simulink model "generic_truck"  (R2025a)
settings: Solver=VariableStepAuto  StartTime=0.0  StopTime=600  FixedStep=0.01  MaxStep=0.001  RelTol=1e-3  EnableMultiTasking=on
libraries: TruckMaker4SL x205, simulink x1
(part 2 of 9)

== system generic_truck/TruckMaker/IPG Vehicle/PowerTrain ==
  note: When replacing the entire powertrain,
      | be sure to disable the IPG powertrain model by using the powertrain
      | model 'Model Manager off' in the vehicle GUI.
  note: <Your model here>
  Sync_In : Inport
  Vhcl.Wheel.PT : Inport  Port=2
  VhclCtrl.PT : Inport  Port=3
  BusCreator : BusCreator  Inputs=99
  Demux : Demux  Outputs=99
      settings: DisplayOption=none
  Gain : Gain
  PowerTrain : S-Function  FunctionName=TM_Sfun  Parameters='PowerTrain'  SFunctionDeploymentMode=off  EnableBusSupport=off
  PowerTrainUpd : S-Function  FunctionName=TM_Sfun  Parameters='PowerTrainUpd'  SFunctionDeploymentMode=off  EnableBusSupport=off
  Sum : Sum  Inputs=|++
  Sync_Out : Outport  VectorParamsAs1DForOutWhenUnconnected=off
  WRR_Trq-drive : Outport  Port=2
  wires:
  Demux/97 -> BusCreator/97  "PT IF WRR4 Trq_Supp2WC"
  Demux/95 -> BusCreator/95  "PT IF WRR4 Trq_B2W"
  Demux/92 -> BusCreator/92  "PT IF WRL4 Trq_BrakeReg_max"
  Demux/88 -> BusCreator/88  "PT IF WRL4 Trq_B2W"
  Demux/89 -> BusCreator/89  "PT IF WRL4 Trq_Drive"
  Demux/86 -> BusCreator/86  "PT IF WRL4 rot"
  Demux/91 -> BusCreator/91  "PT IF WRL4 Trq_BrakeReg"
  Demux/84 -> BusCreator/84  "PT IF WRR3 Trq_BrakeReg"
  Demux/83 -> BusCreator/83  "PT IF WRR3 Trq_Supp2WC"
  Demux/82 -> BusCreator/82  "PT IF WRR3 Trq_Drive"
  Demux/78 -> BusCreator/78  "PT IF WRL3 Trq_BrakeReg_max"
  Demux/87 -> BusCreator/87  "PT IF WRL4 rotv"
  Demux/77 -> BusCreator/77  "PT IF WRL3 Trq_BrakeReg"
  Demux/75 -> BusCreator/75  "PT IF WRL3 Trq_Drive"
  Demux/73 -> BusCreator/73  "PT IF WRL3 rotv"
  Demux/72 -> BusCreator/72  "PT IF WRL3 rot"
  Demux/71 -> BusCreator/71  "PT IF WFR2 Trq_BrakeReg_max"
  Demux/70 -> BusCreator/70  "PT IF WFR2 Trq_BrakeReg"
  Demux/67 -> BusCreator/67  "PT IF WFR2 Trq_B2W"
  Demux/66 -> BusCreator/66  "PT IF WFR2 rotv"
  Demux/80 -> BusCreator/80  "PT IF WRR3 rotv"
  Demux/65 -> BusCreator/65  "PT IF WFR2 rot"
  Demux/76 -> BusCreator/76  "PT IF WRL3 Trq_Supp2WC"
  Demux/63 -> BusCreator/63  "PT IF WFL2 Trq_BrakeReg"
  Demux/74 -> BusCreator/74  "PT IF WRL3 Trq_B2W"
  Demux/69 -> BusCreator/69  "PT IF WFR2 Trq_Supp2WC"
  Demux/58 -> BusCreator/58  "PT IF WFL2 rot"
  Demux/68 -> BusCreator/68  "PT IF WFR2 Trq_Drive"
  Demux/56 -> BusCreator/56  "PT IF WRR2 Trq_BrakeReg"
  Demux/61 -> BusCreator/61  "PT IF WFL2 Trq_Drive"
  Demux/24 -> BusCreator/24  "PT IF WFR rotv"
  BusCreator/1 -> PowerTrainUpd/2
  Demux/20 -> BusCreator/20  "PT IF WFL Trq_Supp2WC"
  Demux/13 -> BusCreator/13  "PT IF Trq_Supp2BdyEng x"
  Demux/99 -> BusCreator/99  "PT IF WRR4 Trq_BrakeReg_max"
  Demux/19 -> BusCreator/19  "PT IF WFL Trq_Drive"
  Demux/33 -> Sum/1, BusCreator/33  "PT IF WRL Trq_Drive"
  Demux/29 -> BusCreator/29  "PT IF WFR Trq_BrakeReg_max"
  Demux/64 -> BusCreator/64  "PT IF WFL2 Trq_BrakeReg_max"
  Demux/57 -> BusCreator/57  "PT IF WRR2 Trq_BrakeReg_max"
  Demux/42 -> BusCreator/42  "PT IF WRR Trq_BrakeReg"
  Demux/16 -> BusCreator/16  "PT IF WFL rot"
  Demux/26 -> BusCreator/26  "PT IF WFR Trq_Drive"
  PowerTrainUpd/1 -> Sync_Out/1
  Demux/93 -> BusCreator/93  "PT IF WRR4 rot"
  Demux/79 -> BusCreator/79  "PT IF WRR3 rot"
  Demux/37 -> BusCreator/37  "PT IF WRR rot"
  Demux/15 -> BusCreator/15  "PT IF DL_iDiff_mean"
  Demux/4 -> BusCreator/4  "PT IF OperationError"
  Demux/59 -> BusCreator/59  "PT IF WFL2 rotv"
  Demux/11 -> BusCreator/11  "PT IF Trq_Supp2Bdy1B y"
  Demux/90 -> BusCreator/90  "PT IF WRL4 Trq_Supp2WC"
  Demux/9 -> BusCreator/9  "PT IF Trq_Supp2Bdy1 z"
  Demux/1 -> BusCreator/1  "PT IF Ignition"
  Demux/98 -> BusCreator/98  "PT IF WRR4 Trq_BrakeReg"
  Demux/17 -> BusCreator/17  "PT IF WFL rotv"
  Sync_In/1 -> PowerTrain/1
  PowerTrain/2 -> Demux/1
  Vhcl.Wheel.PT/1 -> PowerTrain/2
  Demux/14 -> BusCreator/14  "PT IF Trq_Supp2BdyEng y"
  Demux/8 -> BusCreator/8  "PT IF Trq_Supp2Bdy1 y"
  PowerTrain/1 -> PowerTrainUpd/1  "Sync"
  Demux/40 -> Sum/2, BusCreator/40  "PT IF WRR Trq_Drive"
  Demux/12 -> BusCreator/12  "PT IF Trq_Supp2Bdy1B z"
  Demux/2 -> BusCreator/2  "PT IF SelectorCtrl"
  Demux/22 -> BusCreator/22  "PT IF WFL Trq_BrakeReg_max"
  Demux/3 -> BusCreator/3  "PT IF OperationState"
  Demux/10 -> BusCreator/10  "PT IF Trq_Supp2Bdy1B x"
  Demux/18 -> BusCreator/18  "PT IF WFL Trq_B2W"
  Demux/6 -> BusCreator/6  "PT IF Engine_rotv"
  Demux/5 -> BusCreator/5  "PT IF GearNo"
  Demux/27 -> BusCreator/27  "PT IF WFR Trq_Supp2WC"
  Demux/52 -> BusCreator/52  "PT IF WRR2 rotv"
  Demux/28 -> BusCreator/28  "PT IF WFR Trq_BrakeReg"
  Demux/41 -> BusCreator/41  "PT IF WRR Trq_Supp2WC"
  Demux/31 -> BusCreator/31  "PT IF WRL rotv"
  Demux/94 -> BusCreator/94  "PT IF WRR4 rotv"
  Demux/55 -> BusCreator/55  "PT IF WRR2 Trq_Supp2WC"
  Demux/32 -> BusCreator/32  "PT IF WRL Trq_B2W"
  Demux/35 -> BusCreator/35  "PT IF WRL Trq_BrakeReg"
  Demux/25 -> BusCreator/25  "PT IF WFR Trq_B2W"
  Demux/39 -> BusCreator/39  "PT IF WRR Trq_B2W"
  Demux/38 -> BusCreator/38  "PT IF WRR rotv"
  Demux/21 -> BusCreator/21  "PT IF WFL Trq_BrakeReg"
  VhclCtrl.PT/1 -> PowerTrain/3
  Demux/36 -> BusCreator/36  "PT IF WRL Trq_BrakeReg_max"
  Demux/60 -> BusCreator/60  "PT IF WFL2 Trq_B2W"
  Demux/43 -> BusCreator/43  "PT IF WRR Trq_BrakeReg_max"
  Demux/44 -> BusCreator/44  "PT IF WRL2 rot"
  Demux/81 -> BusCreator/81  "PT IF WRR3 Trq_B2W"
  Demux/30 -> BusCreator/30  "PT IF WRL rot"
  Demux/45 -> BusCreator/45  "PT IF WRL2 rotv"
  Demux/23 -> BusCreator/23  "PT IF WFR rot"
  Demux/46 -> BusCreator/46  "PT IF WRL2 Trq_B2W"
  Demux/96 -> BusCreator/96  "PT IF WRR4 Trq_Drive"
  Demux/54 -> BusCreator/54  "PT IF WRR2 Trq_Drive"
  Demux/85 -> BusCreator/85  "PT IF WRR3 Trq_BrakeReg_max"
  Demux/47 -> BusCreator/47  "PT IF WRL2 Trq_Drive"
  Demux/62 -> BusCreator/62  "PT IF WFL2 Trq_Supp2WC"
  Demux/7 -> BusCreator/7  "PT IF Trq_Supp2Bdy1 x"
  Demux/48 -> BusCreator/48  "PT IF WRL2 Trq_Supp2WC"
  Demux/34 -> BusCreator/34  "PT IF WRL Trq_Supp2WC"
  Demux/49 -> BusCreator/49  "PT IF WRL2 Trq_BrakeReg"
  Demux/50 -> BusCreator/50  "PT IF WRL2 Trq_BrakeReg_max"
  Demux/51 -> BusCreator/51  "PT IF WRR2 rot"
  Demux/53 -> BusCreator/53  "PT IF WRR2 Trq_B2W"
  Sum/1 -> Gain/1
  Gain/1 -> WRR_Trq-drive/1

== system generic_truck/TruckMaker/Subsystem1/Measurements from IMU ==
  Acc_x : TruckMaker4SL/Read CM Dict  xname=Sensor.Inertial.Vhcl.VchBdy.Acc_B.x  xsync=off  xstime=Continuous
      settings: SourceProductName=TruckMaker4SL
  Acc_x1 : TruckMaker4SL/Read CM Dict  xname=Vhcl.RL.rotv  xsync=off  xstime=Continuous
      settings: SourceProductName=TruckMaker4SL
  Acc_x2 : TruckMaker4SL/Read CM Dict  xname=Vhcl.RR.rotv  xsync=off  xstime=Continuous
      settings: SourceProductName=TruckMaker4SL
  Acc_x3 : TruckMaker4SL/Read CM Dict  xname=Tr.WheelSpd_ML  xsync=off  xstime=Continuous
      settings: SourceProductName=TruckMaker4SL
  Acc_x4 : TruckMaker4SL/Read CM Dict  xname=Tr.WheelSpd_MR  xsync=off  xstime=Continuous
      settings: SourceProductName=TruckMaker4SL
  Acc_y : TruckMaker4SL/Read CM Dict  xname=Sensor.Inertial.Vhcl.VchBdy.Acc_B.y  xsync=off  xstime=Continuous
      settings: SourceProductName=TruckMaker4SL
  Omega_z : TruckMaker4SL/Read CM Dict  xname=Sensor.Inertial.Vhcl.VchBdy.Omega_B.z  xsync=off  xstime=Continuous
      settings: SourceProductName=TruckMaker4SL
  Vel_x : TruckMaker4SL/Read CM Dict  xname=Sensor.Inertial.Vhcl.VchBdy.Vel_B.x  xsync=off  xstime=Continuous
      settings: SourceProductName=TruckMaker4SL
  Vel_y : TruckMaker4SL/Read CM Dict  xname=Sensor.Inertial.Vhcl.VchBdy.Vel_B.y  xsync=off  xstime=Continuous
      settings: SourceProductName=TruckMaker4SL
  acc_x : Outport
  acc_y : Outport  Port=2
  vel_x : Outport  Port=3
  vel_y : Outport  Port=4
  wz : Outport  Port=5
  omega_rl : Outport  Port=6
  omega_rr : Outport  Port=7
  omega_tr_ML : Outport  Port=8
  omega_tr_MR : Outport  Port=9
  wires:
  Omega_z/1 -> wz/1
  Vel_x/1 -> vel_x/1
  Vel_y/1 -> vel_y/1
  Acc_x/1 -> acc_x/1
  Acc_y/1 -> acc_y/1
  Acc_x2/1 -> omega_rr/1
  Acc_x1/1 -> omega_rl/1
  Acc_x3/1 -> omega_tr_ML/1
  Acc_x4/1 -> omega_tr_MR/1

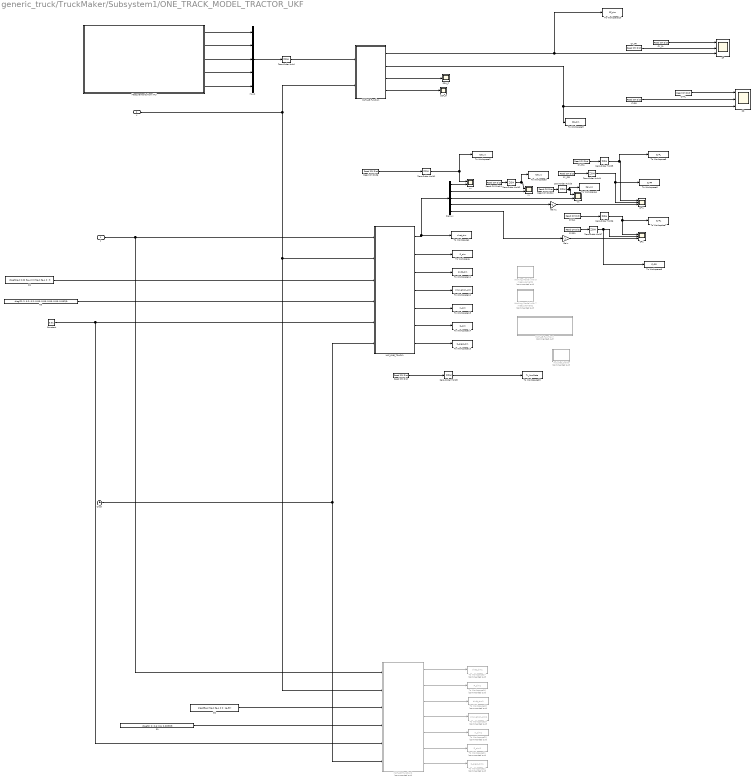
== system generic_truck/TruckMaker/Subsystem1/ONE_TRACK_MODEL_TRACTOR_UKF ==
  z : Inport
  u : Inport  Port=2
  "CF " : Scope  NumInputPorts=3
      settings: ActiveDisplayYMinimum=-12.263034323337607  ActiveDisplayYMaximum=-4.9489164501428942  DataLoggingVariableName=ScopeData23
  CF 1 : Scope  NumInputPorts=3
      settings: ActiveDisplayYMinimum=-10.797860186662938  ActiveDisplayYMaximum=-3.0037046797887497  DataLoggingVariableName=ScopeData30
  CR : Scope  NumInputPorts=3
      settings: ActiveDisplayYMinimum=-11.701585356235972  ActiveDisplayYMaximum=4.5045535239425494  DataLoggingVariableName=ScopeData24
  CR1 : Scope  NumInputPorts=3
      settings: ActiveDisplayYMinimum=-13.474282112558932  ActiveDisplayYMaximum=-8.0648262356989679  DataLoggingVariableName=ScopeData31
  CYRL : TruckMaker4SL/Read CM Dict  xname=CyRL  xsync=off  xstime=Continuous
      settings: SourceProductName=TruckMaker4SL
  CYRL1 : TruckMaker4SL/Read CM Dict  xname=CyRL  xsync=off  xstime=Continuous
      settings: SourceProductName=TruckMaker4SL
  CYRR : TruckMaker4SL/Read CM Dict  xname=CyRR  xsync=off  xstime=Continuous
      settings: SourceProductName=TruckMaker4SL
  CYRR1 : TruckMaker4SL/Read CM Dict  xname=CyRR  xsync=off  xstime=Continuous
      settings: SourceProductName=TruckMaker4SL
  CY_FL : TruckMaker4SL/Read CM Dict  xname=CyFL  xsync=off  xstime=Continuous
      settings: SourceProductName=TruckMaker4SL
  CY_FL1 : TruckMaker4SL/Read CM Dict  xname=CyFL  xsync=off  xstime=Continuous
      settings: SourceProductName=TruckMaker4SL
  CY_FR : TruckMaker4SL/Read CM Dict  xname=CyFR  xsync=off  xstime=Continuous
      settings: SourceProductName=TruckMaker4SL
  CY_FR1 : TruckMaker4SL/Read CM Dict  xname=CyFR  xsync=off  xstime=Continuous
      settings: SourceProductName=TruckMaker4SL
  Clock : Clock
  Constant : Constant  Value=0.01
  Demux : Demux  Outputs=5
  Gain : Gain  Gain=-1
  Gain1 : Gain  Gain=-1
  "Included_trailer " : MATLAB Function  Commented=on  TreatAsAtomicUnit=on
  MATLAB Function : MATLAB Function  TreatAsAtomicUnit=on
  MATLAB Function1 : MATLAB Function  Commented=on  TreatAsAtomicUnit=on
  MATLAB Function2 : MATLAB Function  Commented=on  TreatAsAtomicUnit=on  SystemSampleTime=0.01
  Measurements from IMU : Subsystem  Description=Measurements from IMU Mounted in Vhcl position (3.6; 0.0;1.0)
  Mux2 : Mux  Inputs=5
  Q1 : Constant  Value="diag([2e-2 0.02 3e-4 0 0 5e-2 3e-4 0  ]);"
  Q2 : Constant  Value="diag([5e-2 5e-2 3e-4 0 0  1e-3]);"
  R1 : Constant  Value=diag([2; 2; 0.6; 0.6; 0.005])/3;
  R3 : Constant  Value=diag([2; 2; 0.2; 0.2; 0.05; 0.05; 0.05; 0.05; 0.05])/3;
  Read CM Dict : TruckMaker4SL/Read CM Dict  xname=Tr.YawVel  xsync=off  xstime=Continuous
      settings: SourceProductName=TruckMaker4SL
  Read CM Dict11 : TruckMaker4SL/Read CM Dict  xname=Car.vy  xsync=off  xstime=Continuous
      settings: SourceProductName=TruckMaker4SL
  Read CM Dict12 : TruckMaker4SL/Read CM Dict  xname=Car.YawRate  xsync=off  xstime=Continuous
      settings: SourceProductName=TruckMaker4SL
  Read CM Dict6 : TruckMaker4SL/Read CM Dict  xname=Car.vx  xsync=off  xstime=Continuous
      settings: SourceProductName=TruckMaker4SL
  SSA_F : Scope
      settings: ActiveDisplayYMinimum=-0.046315426334515186  ActiveDisplayYMaximum=0.00321973029301955  DataLoggingVariableName=ScopeData25
  SSA_R : Scope
      settings: ActiveDisplayYMinimum=19.809904868748255  ActiveDisplayYMaximum=19.861105266179973  DataLoggingVariableName=ScopeData26
  To Workspace : ToWorkspace  VariableName=P_sim  SaveFormat=Timeseries  SampleTime=-1
  To Workspace1 : ToWorkspace  VariableName=xhat_sim  SaveFormat=Timeseries  SampleTime=-1
  To Workspace10 : ToWorkspace  VariableName=CF_sim  SaveFormat=Timeseries  SampleTime=-1
  To Workspace11 : ToWorkspace  VariableName=dxdt_sim  SaveFormat=Timeseries  SampleTime=-1
  To Workspace12 : ToWorkspace  VariableName=innovation_sim  SaveFormat=Timeseries  SampleTime=-1
  To Workspace13 : ToWorkspace  VariableName=K_sim  SaveFormat=Timeseries  SampleTime=-1
  To Workspace14 : ToWorkspace  VariableName=S_sim  SaveFormat=Timeseries  SampleTime=-1
  To Workspace15 : ToWorkspace  VariableName=Z_pred_sim  SaveFormat=Timeseries  SampleTime=-1
  To Workspace16 : ToWorkspace  Commented=on  VariableName=P_sim1  SaveFormat=Timeseries  SampleTime=-1
  To Workspace17 : ToWorkspace  Commented=on  VariableName=xhat_sim1  SaveFormat=Timeseries  SampleTime=-1
  To Workspace18 : ToWorkspace  Commented=on  VariableName=dxdt_sim1  SaveFormat=Timeseries  SampleTime=-1
  To Workspace19 : ToWorkspace  Commented=on  VariableName=innovation_sim1  SaveFormat=Timeseries  SampleTime=-1
  To Workspace2 : ToWorkspace  VariableName=Car_vx  SaveFormat=Timeseries  SampleTime=-1
  To Workspace20 : ToWorkspace  Commented=on  VariableName=K_sim1  SaveFormat=Timeseries  SampleTime=-1
  To Workspace21 : ToWorkspace  Commented=on  VariableName=S_sim1  SaveFormat=Timeseries  SampleTime=-1
  To Workspace22 : ToWorkspace  Commented=on  VariableName=Z_pred_sim1  SaveFormat=Timeseries  SampleTime=-1
  To Workspace23 : ToWorkspace  VariableName=Tr_YawRate  SaveFormat=Timeseries  SampleTime=-1
  To Workspace3 : ToWorkspace  VariableName=Car_vy  SaveFormat=Timeseries  SampleTime=-1
  To Workspace4 : ToWorkspace  VariableName=Car_wz  SaveFormat=Timeseries  SampleTime=-1
  To Workspace5 : ToWorkspace  VariableName=CyFL  SaveFormat=Timeseries  SampleTime=-1
  To Workspace6 : ToWorkspace  VariableName=CyFR  SaveFormat=Timeseries  SampleTime=-1
  To Workspace7 : ToWorkspace  VariableName=CyRL  SaveFormat=Timeseries  SampleTime=-1
  To Workspace8 : ToWorkspace  VariableName=CyRR  SaveFormat=Timeseries  SampleTime=-1
  To Workspace9 : ToWorkspace  VariableName=CR_sim  SaveFormat=Timeseries  SampleTime=-1
  UKF_ONE_TRACK1 : MATLAB Function  TreatAsAtomicUnit=on  SystemSampleTime=0.01
  "Working Model with 5 measurements " : MATLAB Function  Commented=on  TreatAsAtomicUnit=on
  Working Model with 7 measurements : MATLAB Function  Commented=on  TreatAsAtomicUnit=on
  Zero-Order Hold{,1..8} (9 alike) : ZeroOrderHold  SampleTime=0.01
  vx : Scope  NumInputPorts=2
      settings: ActiveDisplayYMinimum=15.532965030483135  ActiveDisplayYMaximum=19.510688761225374  DataLoggingVariableName=ScopeData34
  vy : Scope  NumInputPorts=2
      settings: ActiveDisplayYMinimum=-0.016234882238860611  ActiveDisplayYMaximum=0.084455127817541567  DataLoggingVariableName=ScopeData35
  wz : Scope  NumInputPorts=2
      settings: ActiveDisplayYMinimum=-0.21237399330212148  ActiveDisplayYMaximum=0.50990512712526215  DataLoggingVariableName=ScopeData36
  wires:
  MATLAB Function/1(Cf) -> To Workspace10/1, "CF "/3  "Cmptd_Cf"
  Read CM Dict6/1 -> Zero-Order Hold1/1
  CY_FR1/1 -> Zero-Order Hold4/1  "CyFR"
  Demux/1 -> vx/2  "est_vx"
  UKF_ONE_TRACK1/2(P) -> To Workspace/1
  UKF_ONE_TRACK1/1(xhat) -> Demux/1, To Workspace1/1  "State_estimates"
  R3/1 -> UKF_ONE_TRACK1/4(R)
  CYRL1/1 -> Zero-Order Hold6/1  "CyRL"
  Gain/1 -> CR1/3  "est_CR"
  CYRL/1 -> CR/1  "CyRL"
  Constant/1 -> MATLAB Function2/5(Ts), UKF_ONE_TRACK1/5(Ts)
  Read CM Dict12/1 -> Zero-Order Hold3/1
  MATLAB Function/4(alpha_r) -> SSA_R/1
  CYRR1/1 -> Zero-Order Hold7/1  "CyRR"
  CYRR/1 -> CR/2  "CyRR"
  Demux/2 -> vy/2  "est_vy"
  MATLAB Function/2(Cr) -> To Workspace9/1, CR/3  "cmptd_R"
  CY_FL1/1 -> Zero-Order Hold5/1  "CyFL"
  Read CM Dict11/1 -> Zero-Order Hold2/1
  Demux/5 -> Gain/1  "cmptd_R"
  CY_FL/1 -> "CF "/1  "CyFL"
  Demux/3 -> wz/2  "est_wz"
  CY_FR/1 -> "CF "/2  "CyFR"
  MATLAB Function/3(alpha_f) -> SSA_F/1
  Demux/4 -> Gain1/1  "Cmptd_Cf"
  Gain1/1 -> CF 1/3  "Est_CF"
  UKF_ONE_TRACK1/3(dxdt) -> To Workspace11/1
  Q1/1 -> UKF_ONE_TRACK1/3(Q)
  u/1 -> MATLAB Function/2(u), MATLAB Function2/2(u), UKF_ONE_TRACK1/2(u)
  UKF_ONE_TRACK1/4(innovation) -> To Workspace12/1
  UKF_ONE_TRACK1/5(K_out) -> To Workspace13/1
  UKF_ONE_TRACK1/6(S_out) -> To Workspace14/1
  UKF_ONE_TRACK1/7(z_pred_out) -> To Workspace15/1
  z/1 -> MATLAB Function2/1(z), UKF_ONE_TRACK1/1(z)
  Measurements from IMU/1(acc_x) -> Mux2/1
  Measurements from IMU/4(vel_y) -> Mux2/4
  Measurements from IMU/3(vel_x) -> Mux2/3
  Mux2/1 -> Zero-Order Hold/1
  Measurements from IMU/2(acc_y) -> Mux2/2
  Measurements from IMU/5(wz) -> Mux2/5
  Clock/1 -> UKF_ONE_TRACK1/6(data), MATLAB Function2/6(data)
  MATLAB Function2/7(z_pred_out) -> To Workspace22/1
  MATLAB Function2/6(S_out) -> To Workspace21/1
  MATLAB Function2/5(K_out) -> To Workspace20/1
  MATLAB Function2/4(innovation) -> To Workspace19/1
  MATLAB Function2/3(dxdt) -> To Workspace18/1
  MATLAB Function2/1(xhat) -> To Workspace17/1  "State_estimates"
  MATLAB Function2/2(P) -> To Workspace16/1
  R1/1 -> MATLAB Function2/4(R)
  Q2/1 -> MATLAB Function2/3(Q)
  Zero-Order Hold/1 -> MATLAB Function/1(z)
  Zero-Order Hold1/1 -> To Workspace2/1, vx/1
  Zero-Order Hold2/1 -> To Workspace3/1, vy/1
  Zero-Order Hold3/1 -> To Workspace4/1, wz/1
  Zero-Order Hold4/1 -> To Workspace6/1, CF 1/2
  Zero-Order Hold5/1 -> To Workspace5/1, CF 1/1
  Zero-Order Hold6/1 -> To Workspace7/1, CR1/1
  Zero-Order Hold7/1 -> To Workspace8/1, CR1/2
  Read CM Dict/1 -> Zero-Order Hold8/1
  Zero-Order Hold8/1 -> To Workspace23/1

== system generic_truck/TruckMaker/Subsystem1/Subsystem ==
  Ackerman Angle : Subsystem  Commented=on
  Average Steering Angle : Subsystem
  FXh : TruckMaker4SL/Read CM Dict  xname=Tr.Hitch.Frc2Tr.x_1  xsync=off  xstime=Continuous
      settings: SourceProductName=TruckMaker4SL
  FYh : TruckMaker4SL/Read CM Dict  xname=Tr.Hitch.Frc2Tr.y_1  xsync=off  xstime=Continuous
      settings: SourceProductName=TruckMaker4SL
  Trq_RL : TruckMaker4SL/Read CM Dict  xname=Vhcl.RL.Trq_Drive  xsync=off  xstime=Continuous
      settings: SourceProductName=TruckMaker4SL
  Trq_RR : TruckMaker4SL/Read CM Dict  xname=Vhcl.RR.Trq_Drive  xsync=off  xstime=Continuous
      settings: SourceProductName=TruckMaker4SL
  "Average_steering " : Outport
  Trq_T2W_RL : Outport  Port=2
  Trq_T2W_RR : Outport  Port=3
  FXH : Outport  Port=4
  FYH : Outport  Port=5
  wires:
  Trq_RL/1 -> Trq_T2W_RL/1
  Trq_RR/1 -> Trq_T2W_RR/1
  Average Steering Angle/1("Average_steering ") -> "Average_steering "/1
  FXh/1 -> FXH/1
  FYh/1 -> FYH/1

== system generic_truck/TruckMaker/Subsystem1/Subsystem_Noisey Measurements ==
  Acc_x : TruckMaker4SL/Read CM Dict  xname=Vhcl.RL.rotv  xsync=off  xstime=Continuous
      settings: SourceProductName=TruckMaker4SL
  Acc_x1 : TruckMaker4SL/Read CM Dict  xname=Vhcl.RR.rotv  xsync=off  xstime=Continuous
      settings: SourceProductName=TruckMaker4SL
  Acc_x3 : TruckMaker4SL/Read CM Dict  xname=Tr.WheelSpd_ML  xsync=off  xstime=Continuous
      settings: SourceProductName=TruckMaker4SL
  Acc_x4 : TruckMaker4SL/Read CM Dict  xname=Tr.WheelSpd_MR  xsync=off  xstime=Continuous
      settings: SourceProductName=TruckMaker4SL
  Demux : Demux  Outputs=2
  Demux1 : Demux  Outputs=2
  Demux2 : Demux  Outputs=2
  Demux3 : Demux  Outputs=1
  MATLAB Function : MATLAB Function  TreatAsAtomicUnit=on
  MATLAB Function1 : MATLAB Function  TreatAsAtomicUnit=on
  MATLAB Function2 : MATLAB Function  TreatAsAtomicUnit=on
  MATLAB Function3 : MATLAB Function  TreatAsAtomicUnit=on
  Measurements from IMU : Subsystem  Description=Measurements from IMU Mounted in Vhcl position (3.6; 0.0;1.0)
  Mux : Mux  Inputs=3
  Mux1 : Mux  Inputs=3
  Mux2 : Mux  Inputs=5
  Mux3 : Mux  Inputs=3
  Mux5 : Mux  Inputs=2
  Mux6 : Mux  Inputs=2
  Scope : Scope
      settings: ActiveDisplayYMinimum=-5.6580655588196418  ActiveDisplayYMaximum=20.488387754127984  DataLoggingVariableName=ScopeData37
  Out1 : Outport
  wires:
  Mux1/1 -> MATLAB Function2/1(truth)
  Mux2/1 -> Scope/1, Out1/1
  Measurements from IMU/3(acc_z) -> Mux3/3
  Measurements from IMU/2(acc_y) -> Mux3/2
  Measurements from IMU/1(acc_x) -> Mux3/1
  Mux3/1 -> MATLAB Function1/1(acc_true)
  Measurements from IMU/4(vel_x) -> Mux1/1
  Measurements from IMU/5(vel_y) -> Mux1/2
  Measurements from IMU/6(vel_z) -> Mux1/3
  Mux/1 -> MATLAB Function/1(gyro_true)
  Measurements from IMU/7(wx) -> Mux/1
  Measurements from IMU/8(wy) -> Mux/2
  Measurements from IMU/9(wz) -> Mux/3
  Demux/1 -> Mux2/1
  Demux1/1 -> Mux2/2
  Demux2/2 -> Mux2/3
  MATLAB Function1/1(acc_meas) -> Demux/1
  MATLAB Function2/1(vel_meas) -> Demux1/1
  MATLAB Function/1(gyro_meas) -> Demux2/1
  MATLAB Function3/1(vel_meas) -> Demux3/1
  Acc_x1/1 -> Mux5/2
  Acc_x/1 -> Mux5/1
  Mux5/1 -> MATLAB Function3/1(truth)
  Demux3/1 -> Mux2/4
  Mux6/1 -> Mux2/5
  Acc_x3/1 -> Mux6/1
  Acc_x4/1 -> Mux6/2

== system generic_truck/TruckMaker/Subsystem1/Subsystem_Noisey Measurements _NAN ==
  Acc_x : TruckMaker4SL/Read CM Dict  xname=Vhcl.RL.rotv  xsync=off  xstime=Continuous
      settings: SourceProductName=TruckMaker4SL
  Acc_x1 : TruckMaker4SL/Read CM Dict  xname=Vhcl.RR.rotv  xsync=off  xstime=Continuous
      settings: SourceProductName=TruckMaker4SL
  Acc_x3 : TruckMaker4SL/Read CM Dict  xname=Tr.WheelSpd_ML  xsync=off  xstime=Continuous
      settings: SourceProductName=TruckMaker4SL
  Acc_x4 : TruckMaker4SL/Read CM Dict  xname=Tr.WheelSpd_MR  xsync=off  xstime=Continuous
      settings: SourceProductName=TruckMaker4SL
  Demux : Demux  Outputs=2
  Demux1 : Demux  Outputs=2
  Demux2 : Demux  Outputs=2
  Demux3 : Demux  Outputs=1
  MATLAB Function : MATLAB Function  TreatAsAtomicUnit=on
  MATLAB Function1 : MATLAB Function  TreatAsAtomicUnit=on
  MATLAB Function2 : MATLAB Function  TreatAsAtomicUnit=on
  MATLAB Function3 : MATLAB Function  TreatAsAtomicUnit=on
  Manual Switch : ManualSwitch  CurrentSetting=0
  Measurements from IMU : Subsystem  Description=Measurements from IMU Mounted in Vhcl position (3.6; 0.0;1.0)
  Mux : Mux  Inputs=3
  Mux1 : Mux  Inputs=3
  Mux2 : Mux  Inputs=5
  Mux3 : Mux  Inputs=3
  Mux4 : Mux  Inputs=2
  Mux5 : Mux  Inputs=2
  Mux6 : Mux  Inputs=2
  NaN : Constant  Value=NaN  OutDataTypeStr=Inherit: Inherit via back propagation
  Scope : Scope
      settings: ActiveDisplayYMinimum=-12.833093805155979  ActiveDisplayYMaximum=56.830382589328167  DataLoggingVariableName=ScopeData37
  Out1 : Outport
  wires:
  MATLAB Function/1(gyro_meas) -> Demux2/1
  MATLAB Function2/1(vel_meas) -> Demux1/1
  MATLAB Function1/1(acc_meas) -> Demux/1
  Demux2/2 -> Mux2/3
  Demux/1 -> Mux2/1
  Measurements from IMU/9(wz) -> Mux/3
  Measurements from IMU/8(wy) -> Mux/2
  Measurements from IMU/7(wx) -> Mux/1
  Mux/1 -> MATLAB Function/1(gyro_true)
  Measurements from IMU/6(vel_z) -> Mux1/3
  Measurements from IMU/5(vel_y) -> Mux1/2
  Measurements from IMU/4(vel_x) -> Mux1/1
  Mux3/1 -> MATLAB Function1/1(acc_true)
  Measurements from IMU/1(acc_x) -> Mux3/1
  Measurements from IMU/2(acc_y) -> Mux3/2
  Measurements from IMU/3(acc_z) -> Mux3/3
  Mux2/1 -> Scope/1, Out1/1
  Mux1/1 -> MATLAB Function2/1(truth)
  NaN/1 -> Mux4/1, Mux4/2
  Mux4/1 -> Manual Switch/2
  Demux1/1 -> Manual Switch/1
  Manual Switch/1 -> Mux2/2
  Mux5/1 -> MATLAB Function3/1(truth)
  MATLAB Function3/1(vel_meas) -> Demux3/1
  Acc_x/1 -> Mux5/1
  Acc_x1/1 -> Mux5/2
  Demux3/1 -> Mux2/4
  Acc_x3/1 -> Mux6/1
  Acc_x4/1 -> Mux6/2
  Mux6/1 -> Mux2/5

== system generic_truck/TruckMaker/Tractor_Subsystem /Measurements from IMU ==
  Acc_x : TruckMaker4SL/Read CM Dict  xname=Sensor.Inertial.Vhcl.VchBdy.Acc_B.x  xsync=off  xstime=Continuous
      settings: SourceProductName=TruckMaker4SL
  Acc_x1 : TruckMaker4SL/Read CM Dict  xname=Vhcl.RL.rotv  xsync=off  xstime=Continuous
      settings: SourceProductName=TruckMaker4SL
  Acc_x2 : TruckMaker4SL/Read CM Dict  xname=Vhcl.RR.rotv  xsync=off  xstime=Continuous
      settings: SourceProductName=TruckMaker4SL
  Acc_y : TruckMaker4SL/Read CM Dict  xname=Sensor.Inertial.Vhcl.VchBdy.Acc_B.y  xsync=off  xstime=Continuous
      settings: SourceProductName=TruckMaker4SL
  Omega_z : TruckMaker4SL/Read CM Dict  xname=Sensor.Inertial.Vhcl.VchBdy.Omega_B.z  xsync=off  xstime=Continuous
      settings: SourceProductName=TruckMaker4SL
  Vel_x : TruckMaker4SL/Read CM Dict  xname=Sensor.Inertial.Vhcl.VchBdy.Vel_B.x  xsync=off  xstime=Continuous
      settings: SourceProductName=TruckMaker4SL
  Vel_y : TruckMaker4SL/Read CM Dict  xname=Sensor.Inertial.Vhcl.VchBdy.Vel_B.y  xsync=off  xstime=Continuous
      settings: SourceProductName=TruckMaker4SL
  acc_x : Outport
  acc_y : Outport  Port=2
  vel_x : Outport  Port=3
  vel_y : Outport  Port=4
  wz : Outport  Port=5
  omega_rl : Outport  Port=6
  omega_rr : Outport  Port=7
  wires:
  Acc_y/1 -> acc_y/1
  Acc_x/1 -> acc_x/1
  Vel_y/1 -> vel_y/1
  Vel_x/1 -> vel_x/1
  Omega_z/1 -> wz/1
  Acc_x1/1 -> omega_rl/1
  Acc_x2/1 -> omega_rr/1

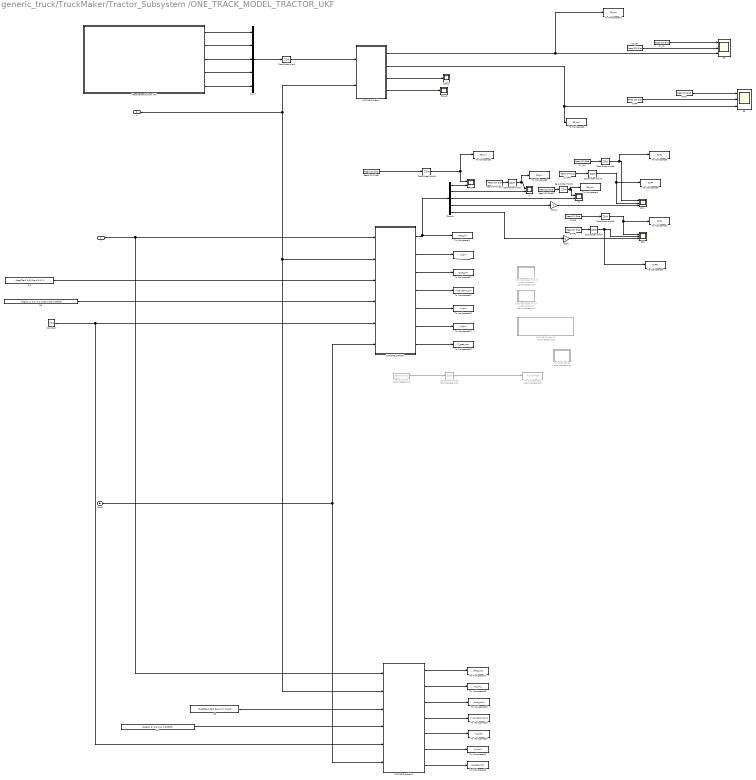
== system generic_truck/TruckMaker/Tractor_Subsystem /ONE_TRACK_MODEL_TRACTOR_UKF ==
  z : Inport
  u : Inport  Port=2
  "CF " : Scope  NumInputPorts=3
      settings: ActiveDisplayYMinimum=-12.263034323337607  ActiveDisplayYMaximum=-4.9489164501428942  DataLoggingVariableName=ScopeData23
  CF 1 : Scope  NumInputPorts=3
      settings: ActiveDisplayYMinimum=-10.797860186662938  ActiveDisplayYMaximum=-3.0037046797887497  DataLoggingVariableName=ScopeData30
  CR : Scope  NumInputPorts=3
      settings: ActiveDisplayYMinimum=-11.701585356235972  ActiveDisplayYMaximum=4.5045535239425494  DataLoggingVariableName=ScopeData24
  CR1 : Scope  NumInputPorts=3
      settings: ActiveDisplayYMinimum=-13.474282112558932  ActiveDisplayYMaximum=-8.0648262356989679  DataLoggingVariableName=ScopeData31
  CYRL : TruckMaker4SL/Read CM Dict  xname=CyRL  xsync=off  xstime=Continuous
      settings: SourceProductName=TruckMaker4SL
  CYRL1 : TruckMaker4SL/Read CM Dict  xname=CyRL  xsync=off  xstime=Continuous
      settings: SourceProductName=TruckMaker4SL
  CYRR : TruckMaker4SL/Read CM Dict  xname=CyRR  xsync=off  xstime=Continuous
      settings: SourceProductName=TruckMaker4SL
  CYRR1 : TruckMaker4SL/Read CM Dict  xname=CyRR  xsync=off  xstime=Continuous
      settings: SourceProductName=TruckMaker4SL
  CY_FL : TruckMaker4SL/Read CM Dict  xname=CyFL  xsync=off  xstime=Continuous
      settings: SourceProductName=TruckMaker4SL
  CY_FL1 : TruckMaker4SL/Read CM Dict  xname=CyFL  xsync=off  xstime=Continuous
      settings: SourceProductName=TruckMaker4SL
  CY_FR : TruckMaker4SL/Read CM Dict  xname=CyFR  xsync=off  xstime=Continuous
      settings: SourceProductName=TruckMaker4SL
  CY_FR1 : TruckMaker4SL/Read CM Dict  xname=CyFR  xsync=off  xstime=Continuous
      settings: SourceProductName=TruckMaker4SL
  Clock : Clock
  Constant : Constant  Value=0.01
  Demux : Demux  Outputs=5
  Gain : Gain  Gain=-1
  Gain1 : Gain  Gain=-1
  "Included_trailer " : MATLAB Function  Commented=on  TreatAsAtomicUnit=on
  MATLAB Function : MATLAB Function  TreatAsAtomicUnit=on
  MATLAB Function1 : MATLAB Function  Commented=on  TreatAsAtomicUnit=on
  MATLAB Function2 : MATLAB Function  TreatAsAtomicUnit=on  SystemSampleTime=0.01
  Measurements from IMU : Subsystem  Description=Measurements from IMU Mounted in Vhcl position (3.6; 0.0;1.0)
  Mux2 : Mux  Inputs=5
  Q1 : Constant  Value="diag([2e-2 0.02 3e-4 0 0  ]);"
  Q2 : Constant  Value="diag([5e-2 5e-2 3e-4 0 0  1e-3]);"
  R1 : Constant  Value=diag([2; 2; 0.6; 0.6; 0.005])/3;
  R3 : Constant  Value=diag([2; 2; 0.2; 0.2; 0.05; 0.05; 0.05])/3;
  Read CM Dict : TruckMaker4SL/Read CM Dict  Commented=on  xname=Tr.YawVel  xsync=off  xstime=Continuous
      settings: SourceProductName=TruckMaker4SL
  Read CM Dict11 : TruckMaker4SL/Read CM Dict  xname=Car.vy  xsync=off  xstime=Continuous
      settings: SourceProductName=TruckMaker4SL
  Read CM Dict12 : TruckMaker4SL/Read CM Dict  xname=Car.YawRate  xsync=off  xstime=Continuous
      settings: SourceProductName=TruckMaker4SL
  Read CM Dict6 : TruckMaker4SL/Read CM Dict  xname=Car.vx  xsync=off  xstime=Continuous
      settings: SourceProductName=TruckMaker4SL
  SSA_F : Scope
      settings: ActiveDisplayYMinimum=-0.046315426334515186  ActiveDisplayYMaximum=0.00321973029301955  DataLoggingVariableName=ScopeData25
  SSA_R : Scope
      settings: ActiveDisplayYMinimum=19.809904868748255  ActiveDisplayYMaximum=19.861105266179973  DataLoggingVariableName=ScopeData26
  To Workspace : ToWorkspace  VariableName=P_sim  SaveFormat=Timeseries  SampleTime=-1
  To Workspace1 : ToWorkspace  VariableName=xhat_sim  SaveFormat=Timeseries  SampleTime=-1
  To Workspace10 : ToWorkspace  VariableName=CF_sim  SaveFormat=Timeseries  SampleTime=-1
  To Workspace11 : ToWorkspace  VariableName=dxdt_sim  SaveFormat=Timeseries  SampleTime=-1
  To Workspace12 : ToWorkspace  VariableName=innovation_sim  SaveFormat=Timeseries  SampleTime=-1
  To Workspace13 : ToWorkspace  VariableName=K_sim  SaveFormat=Timeseries  SampleTime=-1
  To Workspace14 : ToWorkspace  VariableName=S_sim  SaveFormat=Timeseries  SampleTime=-1
  To Workspace15 : ToWorkspace  VariableName=Z_pred_sim  SaveFormat=Timeseries  SampleTime=-1
  To Workspace16 : ToWorkspace  VariableName=P_sim1  SaveFormat=Timeseries  SampleTime=-1
  To Workspace17 : ToWorkspace  VariableName=xhat_sim1  SaveFormat=Timeseries  SampleTime=-1
  To Workspace18 : ToWorkspace  VariableName=dxdt_sim1  SaveFormat=Timeseries  SampleTime=-1
  To Workspace19 : ToWorkspace  VariableName=innovation_sim1  SaveFormat=Timeseries  SampleTime=-1
  To Workspace2 : ToWorkspace  VariableName=Car_vx  SaveFormat=Timeseries  SampleTime=-1
  To Workspace20 : ToWorkspace  VariableName=K_sim1  SaveFormat=Timeseries  SampleTime=-1
  To Workspace21 : ToWorkspace  VariableName=S_sim1  SaveFormat=Timeseries  SampleTime=-1
  To Workspace22 : ToWorkspace  VariableName=Z_pred_sim1  SaveFormat=Timeseries  SampleTime=-1
  To Workspace23 : ToWorkspace  Commented=on  VariableName=Tr_YawRate  SaveFormat=Timeseries  SampleTime=-1
  To Workspace3 : ToWorkspace  VariableName=Car_vy  SaveFormat=Timeseries  SampleTime=-1
  To Workspace4 : ToWorkspace  VariableName=Car_wz  SaveFormat=Timeseries  SampleTime=-1
  To Workspace5 : ToWorkspace  VariableName=CyFL  SaveFormat=Timeseries  SampleTime=-1
  To Workspace6 : ToWorkspace  VariableName=CyFR  SaveFormat=Timeseries  SampleTime=-1
  To Workspace7 : ToWorkspace  VariableName=CyRL  SaveFormat=Timeseries  SampleTime=-1
  To Workspace8 : ToWorkspace  VariableName=CyRR  SaveFormat=Timeseries  SampleTime=-1
  To Workspace9 : ToWorkspace  VariableName=CR_sim  SaveFormat=Timeseries  SampleTime=-1
  UKF_ONE_TRACK1 : MATLAB Function  TreatAsAtomicUnit=on  SystemSampleTime=0.01
  "Working Model with 5 measurements " : MATLAB Function  Commented=on  TreatAsAtomicUnit=on
  Working Model with 7 measurements : MATLAB Function  Commented=on  TreatAsAtomicUnit=on
  Zero-Order Hold{,1..7} (8 alike) : ZeroOrderHold  SampleTime=0.01
  Zero-Order Hold8 : ZeroOrderHold  Commented=on  SampleTime=0.01
  vx : Scope  NumInputPorts=2
      settings: ActiveDisplayYMinimum=15.532965030483135  ActiveDisplayYMaximum=19.510688761225374  DataLoggingVariableName=ScopeData34
  vy : Scope  NumInputPorts=2
      settings: ActiveDisplayYMinimum=-0.016234882238860611  ActiveDisplayYMaximum=0.084455127817541567  DataLoggingVariableName=ScopeData35
  wz : Scope  NumInputPorts=2
      settings: ActiveDisplayYMinimum=-0.21237399330212148  ActiveDisplayYMaximum=0.50990512712526215  DataLoggingVariableName=ScopeData36
  wires:
  Zero-Order Hold8/1 -> To Workspace23/1
  Read CM Dict/1 -> Zero-Order Hold8/1
  Zero-Order Hold7/1 -> CR1/2, To Workspace8/1
  Zero-Order Hold6/1 -> CR1/1, To Workspace7/1
  Zero-Order Hold5/1 -> CF 1/1, To Workspace5/1
  Zero-Order Hold4/1 -> CF 1/2, To Workspace6/1
  Zero-Order Hold3/1 -> wz/1, To Workspace4/1
  Zero-Order Hold2/1 -> vy/1, To Workspace3/1
  Zero-Order Hold1/1 -> vx/1, To Workspace2/1
  Zero-Order Hold/1 -> MATLAB Function/1(z)
  Q2/1 -> MATLAB Function2/3(Q)
  R1/1 -> MATLAB Function2/4(R)
  MATLAB Function2/2(P) -> To Workspace16/1
  MATLAB Function2/1(xhat) -> To Workspace17/1  "State_estimates"
  MATLAB Function2/3(dxdt) -> To Workspace18/1
  MATLAB Function2/4(innovation) -> To Workspace19/1
  MATLAB Function2/5(K_out) -> To Workspace20/1
  MATLAB Function2/6(S_out) -> To Workspace21/1
  MATLAB Function2/7(z_pred_out) -> To Workspace22/1
  Clock/1 -> MATLAB Function2/6(data), UKF_ONE_TRACK1/6(data)
  Measurements from IMU/5(wz) -> Mux2/5
  Measurements from IMU/2(acc_y) -> Mux2/2
  Mux2/1 -> Zero-Order Hold/1
  Measurements from IMU/3(vel_x) -> Mux2/3
  Measurements from IMU/4(vel_y) -> Mux2/4
  Measurements from IMU/1(acc_x) -> Mux2/1
  z/1 -> UKF_ONE_TRACK1/1(z), MATLAB Function2/1(z)
  UKF_ONE_TRACK1/7(z_pred_out) -> To Workspace15/1
  UKF_ONE_TRACK1/6(S_out) -> To Workspace14/1
  UKF_ONE_TRACK1/5(K_out) -> To Workspace13/1
  UKF_ONE_TRACK1/4(innovation) -> To Workspace12/1
  u/1 -> UKF_ONE_TRACK1/2(u), MATLAB Function2/2(u), MATLAB Function/2(u)
  Q1/1 -> UKF_ONE_TRACK1/3(Q)
  UKF_ONE_TRACK1/3(dxdt) -> To Workspace11/1
  Gain1/1 -> CF 1/3  "Est_CF"
  Demux/4 -> Gain1/1  "Cmptd_Cf"
  MATLAB Function/3(alpha_f) -> SSA_F/1
  CY_FR/1 -> "CF "/2  "CyFR"
  Demux/3 -> wz/2  "est_wz"
  CY_FL/1 -> "CF "/1  "CyFL"
  Demux/5 -> Gain/1  "cmptd_R"
  Read CM Dict11/1 -> Zero-Order Hold2/1
  CY_FL1/1 -> Zero-Order Hold5/1  "CyFL"
  MATLAB Function/2(Cr) -> CR/3, To Workspace9/1  "cmptd_R"
  Demux/2 -> vy/2  "est_vy"
  CYRR/1 -> CR/2  "CyRR"
  CYRR1/1 -> Zero-Order Hold7/1  "CyRR"
  MATLAB Function/4(alpha_r) -> SSA_R/1
  Read CM Dict12/1 -> Zero-Order Hold3/1
  Constant/1 -> UKF_ONE_TRACK1/5(Ts), MATLAB Function2/5(Ts)
  CYRL/1 -> CR/1  "CyRL"
  Gain/1 -> CR1/3  "est_CR"
  CYRL1/1 -> Zero-Order Hold6/1  "CyRL"
  R3/1 -> UKF_ONE_TRACK1/4(R)
  UKF_ONE_TRACK1/1(xhat) -> To Workspace1/1, Demux/1  "State_estimates"
  UKF_ONE_TRACK1/2(P) -> To Workspace/1
  Demux/1 -> vx/2  "est_vx"
  CY_FR1/1 -> Zero-Order Hold4/1  "CyFR"
  Read CM Dict6/1 -> Zero-Order Hold1/1
  MATLAB Function/1(Cf) -> "CF "/3, To Workspace10/1  "Cmptd_Cf"

== system generic_truck/TruckMaker/Tractor_Subsystem /Subsystem ==
  Ackerman Angle : Subsystem  Commented=on
  Average Steering Angle : Subsystem
  "Bromsmoment fram " : Subsystem
  Bromsmoment rear 1 : Subsystem
  Scope1 : Scope
      settings: ActiveDisplayYMinimum=-1813.6997625686197  ActiveDisplayYMaximum=16323.297863117581  DataLoggingVariableName=ScopeData40
  Scope2 : Scope
      settings: ActiveDisplayYMinimum=-1  ActiveDisplayYMaximum=1  DataLoggingVariableName=ScopeData41
  Trq_RL : TruckMaker4SL/Read CM Dict  xname=Vhcl.RL.Trq_Drive  xsync=off  xstime=Continuous
      settings: SourceProductName=TruckMaker4SL
  Trq_RR : TruckMaker4SL/Read CM Dict  xname=Vhcl.RR.Trq_Drive  xsync=off  xstime=Continuous
      settings: SourceProductName=TruckMaker4SL
  "Average_steering " : Outport
  Trq_T2W_RL : Outport  Port=2
  Trq_T2W_RR : Outport  Port=3
  TBF : Outport  Port=4
  TBR : Outport  Port=5
  wires:
  Average Steering Angle/1("Average_steering ") -> "Average_steering "/1
  Trq_RR/1 -> Trq_T2W_RR/1
  Trq_RL/1 -> Trq_T2W_RL/1
  "Bromsmoment fram "/1("Average_Bromsmomet ") -> Scope1/1, TBF/1
  Bromsmoment rear 1/1("Average_Bromsmomet ") -> Scope2/1, TBR/1

== system generic_truck/TruckMaker/Tractor_Subsystem /Subsystem_Noisey Measurements ==
  Acc_x : TruckMaker4SL/Read CM Dict  xname=Vhcl.RL.rotv  xsync=off  xstime=Continuous
      settings: SourceProductName=TruckMaker4SL
  Acc_x1 : TruckMaker4SL/Read CM Dict  xname=Vhcl.RR.rotv  xsync=off  xstime=Continuous
      settings: SourceProductName=TruckMaker4SL
  Demux : Demux  Outputs=2
  Demux1 : Demux  Outputs=2
  Demux2 : Demux  Outputs=2
  Demux3 : Demux  Outputs=1
  MATLAB Function : MATLAB Function  TreatAsAtomicUnit=on
  MATLAB Function1 : MATLAB Function  TreatAsAtomicUnit=on
  MATLAB Function2 : MATLAB Function  TreatAsAtomicUnit=on
  MATLAB Function3 : MATLAB Function  TreatAsAtomicUnit=on
  Measurements from IMU : Subsystem  Description=Measurements from IMU Mounted in Vhcl position (3.6; 0.0;1.0)
  Mux : Mux  Inputs=3
  Mux1 : Mux  Inputs=3
  Mux2 : Mux
  Mux3 : Mux  Inputs=3
  Mux5 : Mux  Inputs=2
  Scope : Scope
      settings: ActiveDisplayYMinimum=-5.6580655588196418  ActiveDisplayYMaximum=20.488387754127984  DataLoggingVariableName=ScopeData37
  Out1 : Outport
  wires:
  MATLAB Function/1(gyro_meas) -> Demux2/1
  MATLAB Function2/1(vel_meas) -> Demux1/1
  MATLAB Function1/1(acc_meas) -> Demux/1
  Demux2/2 -> Mux2/3
  Demux1/1 -> Mux2/2
  Demux/1 -> Mux2/1
  Measurements from IMU/9(wz) -> Mux/3
  Measurements from IMU/8(wy) -> Mux/2
  Measurements from IMU/7(wx) -> Mux/1
  Mux/1 -> MATLAB Function/1(gyro_true)
  Measurements from IMU/6(vel_z) -> Mux1/3
  Measurements from IMU/5(vel_y) -> Mux1/2
  Measurements from IMU/4(vel_x) -> Mux1/1
  Mux3/1 -> MATLAB Function1/1(acc_true)
  Measurements from IMU/1(acc_x) -> Mux3/1
  Measurements from IMU/2(acc_y) -> Mux3/2
  Measurements from IMU/3(acc_z) -> Mux3/3
  Mux2/1 -> Out1/1, Scope/1
  Mux1/1 -> MATLAB Function2/1(truth)
  Acc_x/1 -> Mux5/1
  Acc_x1/1 -> Mux5/2
  Mux5/1 -> MATLAB Function3/1(truth)
  Demux3/1 -> Mux2/4
  MATLAB Function3/1(vel_meas) -> Demux3/1

== system generic_truck/TruckMaker/Tractor_Subsystem /Subsystem_Noisey Measurements _NAN ==
  Acc_x : TruckMaker4SL/Read CM Dict  xname=Vhcl.RL.rotv  xsync=off  xstime=Continuous
      settings: SourceProductName=TruckMaker4SL
  Acc_x1 : TruckMaker4SL/Read CM Dict  xname=Vhcl.RR.rotv  xsync=off  xstime=Continuous
      settings: SourceProductName=TruckMaker4SL
  Demux : Demux  Outputs=2
  Demux1 : Demux  Outputs=2
  Demux2 : Demux  Outputs=2
  Demux3 : Demux  Outputs=1
  MATLAB Function : MATLAB Function  TreatAsAtomicUnit=on
  MATLAB Function1 : MATLAB Function  TreatAsAtomicUnit=on
  MATLAB Function2 : MATLAB Function  TreatAsAtomicUnit=on
  MATLAB Function3 : MATLAB Function  TreatAsAtomicUnit=on
  Manual Switch : ManualSwitch  CurrentSetting=0
  Measurements from IMU : Subsystem  Description=Measurements from IMU Mounted in Vhcl position (3.6; 0.0;1.0)
  Mux : Mux  Inputs=3
  Mux1 : Mux  Inputs=3
  Mux2 : Mux
  Mux3 : Mux  Inputs=3
  Mux4 : Mux  Inputs=2
  Mux5 : Mux  Inputs=2
  NaN : Constant  Value=NaN  OutDataTypeStr=Inherit: Inherit via back propagation
  Scope : Scope
      settings: ActiveDisplayYMinimum=-12.833093805155979  ActiveDisplayYMaximum=56.830382589328167  DataLoggingVariableName=ScopeData37
  Out1 : Outport
  wires:
  Manual Switch/1 -> Mux2/2
  Demux1/1 -> Manual Switch/1
  Mux4/1 -> Manual Switch/2
  NaN/1 -> Mux4/2, Mux4/1
  Mux1/1 -> MATLAB Function2/1(truth)
  Mux2/1 -> Out1/1, Scope/1
  Measurements from IMU/3(acc_z) -> Mux3/3
  Measurements from IMU/2(acc_y) -> Mux3/2
  Measurements from IMU/1(acc_x) -> Mux3/1
  Mux3/1 -> MATLAB Function1/1(acc_true)
  Measurements from IMU/4(vel_x) -> Mux1/1
  Measurements from IMU/5(vel_y) -> Mux1/2
  Measurements from IMU/6(vel_z) -> Mux1/3
  Mux/1 -> MATLAB Function/1(gyro_true)
  Measurements from IMU/7(wx) -> Mux/1
  Measurements from IMU/8(wy) -> Mux/2
  Measurements from IMU/9(wz) -> Mux/3
  Demux/1 -> Mux2/1
  Demux2/2 -> Mux2/3
  MATLAB Function1/1(acc_meas) -> Demux/1
  MATLAB Function2/1(vel_meas) -> Demux1/1
  MATLAB Function/1(gyro_meas) -> Demux2/1
  Acc_x/1 -> Mux5/1
  Acc_x1/1 -> Mux5/2
  Mux5/1 -> MATLAB Function3/1(truth)
  Demux3/1 -> Mux2/4
  MATLAB Function3/1(vel_meas) -> Demux3/1

== system generic_truck/TruckMaker/VehicleControl/CreateBus Vhcl.Misc ==
  In1 : Inport
  Bus Creator5 : BusCreator  Inputs=11
  Demux5 : Demux  Outputs=11
      settings: DisplayOption=none
  Out1 : Outport  VectorParamsAs1DForOutWhenUnconnected=off
  wires:
  Demux5/11 -> Bus Creator5/11  "Vhcl Wind_vel_0 z"
  Demux5/10 -> Bus Creator5/10  "Vhcl Wind_vel_0 y"
  Demux5/9 -> Bus Creator5/9  "Vhcl Wind_vel_0 x"
  Demux5/8 -> Bus Creator5/8  "Vhcl DL2BdyEng y"
  Demux5/7 -> Bus Creator5/7  "Vhcl DL2BdyEng x"
  Demux5/6 -> Bus Creator5/6  "Vhcl TrqDL2Bdy1B z"
  Demux5/5 -> Bus Creator5/5  "Vhcl TrqDL2Bdy1B y"
  Demux5/4 -> Bus Creator5/4  "Vhcl TrqDL2Bdy1B x"
  Demux5/3 -> Bus Creator5/3  "Vhcl Trq_DL2Bdy1 z"
  In1/1 -> Demux5/1
  Bus Creator5/1 -> Out1/1
  Demux5/2 -> Bus Creator5/2  "Vhcl Trq_DL2Bdy1 y"
  Demux5/1 -> Bus Creator5/1  "Vhcl Trq_DL2Bdy1 x"

== system generic_truck/TruckMaker/VehicleControl/CreateBus Vhcl.Wheel.In ==
  In1 : Inport
  Bus Creator1 : BusCreator  Inputs=36
  Demux1 : Demux  Outputs=36
      settings: DisplayOption=none
  Out1 : Outport  VectorParamsAs1DForOutWhenUnconnected=off
  wires:
  Demux1/36 -> Bus Creator1/36  "Vhcl Wheel RR4 rotv"
  Demux1/35 -> Bus Creator1/35  "Vhcl Wheel RR4 Trq_DL2WC"
  Demux1/34 -> Bus Creator1/34  "Vhcl Wheel RR4 Trq_B2WC"
  Demux1/33 -> Bus Creator1/33  "Vhcl Wheel RL4 rotv"
  Demux1/32 -> Bus Creator1/32  "Vhcl Wheel RL4 Trq_DL2WC"
  Demux1/31 -> Bus Creator1/31  "Vhcl Wheel RL4 Trq_B2WC"
  Demux1/30 -> Bus Creator1/30  "Vhcl Wheel RR3 rotv"
  Demux1/29 -> Bus Creator1/29  "Vhcl Wheel RR3 Trq_DL2WC"
  Demux1/28 -> Bus Creator1/28  "Vhcl Wheel RR3 Trq_B2WC"
  Demux1/27 -> Bus Creator1/27  "Vhcl Wheel RL3 rotv"
  Demux1/26 -> Bus Creator1/26  "Vhcl Wheel RL3 Trq_DL2WC"
  Demux1/25 -> Bus Creator1/25  "Vhcl Wheel RL3 Trq_B2WC"
  Demux1/12 -> Bus Creator1/12  "Vhcl Wheel RR rotv"
  Demux1/11 -> Bus Creator1/11  "Vhcl Wheel RR Trq_DL2WC"
  Demux1/10 -> Bus Creator1/10  "Vhcl Wheel RR Trq_B2WC"
  Demux1/9 -> Bus Creator1/9  "Vhcl Wheel RL rotv"
  Demux1/8 -> Bus Creator1/8  "Vhcl Wheel RL Trq_DL2WC"
  Demux1/7 -> Bus Creator1/7  "Vhcl Wheel RL Trq_B2WC"
  Demux1/6 -> Bus Creator1/6  "Vhcl Wheel FR rotv"
  Demux1/5 -> Bus Creator1/5  "Vhcl Wheel FR Trq_DL2WC"
  Demux1/4 -> Bus Creator1/4  "Vhcl Wheel FR Trq_B2WC"
  Demux1/3 -> Bus Creator1/3  "Vhcl Wheel FL rotv"
  Demux1/2 -> Bus Creator1/2  "Vhcl Wheel FL Trq_DL2WC"
  Demux1/1 -> Bus Creator1/1  "Vhcl Wheel FL Trq_B2WC"
  Bus Creator1/1 -> Out1/1
  In1/1 -> Demux1/1
  Demux1/24 -> Bus Creator1/24  "Vhcl Wheel FR2 rotv"
  Demux1/23 -> Bus Creator1/23  "Vhcl Wheel FR2 Trq_DL2WC"
  Demux1/22 -> Bus Creator1/22  "Vhcl Wheel FR2 Trq_B2WC"
  Demux1/21 -> Bus Creator1/21  "Vhcl Wheel FL2 rotv"
  Demux1/20 -> Bus Creator1/20  "Vhcl Wheel FL2 Trq_DL2WC"
  Demux1/19 -> Bus Creator1/19  "Vhcl Wheel FL2 Trq_B2WC"
  Demux1/18 -> Bus Creator1/18  "Vhcl Wheel RR2 rotv"
  Demux1/17 -> Bus Creator1/17  "Vhcl Wheel RR2 Trq_DL2WC"
  Demux1/16 -> Bus Creator1/16  "Vhcl Wheel RR2 Trq_B2WC"
  Demux1/15 -> Bus Creator1/15  "Vhcl Wheel RL2 rotv"
  Demux1/14 -> Bus Creator1/14  "Vhcl Wheel RL2 Trq_DL2WC"
  Demux1/13 -> Bus Creator1/13  "Vhcl Wheel RL2 Trq_B2WC"

== system generic_truck/TruckMaker/VehicleControl/CreateBus VhclCtrl ==
  In : Inport
  BusCreator : BusCreator  Inputs=29
  Demux : Demux  Outputs=29
      settings: DisplayOption=none
  Out : Outport  VectorParamsAs1DForOutWhenUnconnected=off
  wires:
  Demux/29 -> BusCreator/29  "VhclCtrl Lights Reverse"
  Demux/28 -> BusCreator/28  "VhclCtrl Lights Brake"
  Demux/27 -> BusCreator/27  "VhclCtrl Lights FogRear"
  Demux/26 -> BusCreator/26  "VhclCtrl Lights FogFrontR"
  Demux/25 -> BusCreator/25  "VhclCtrl Lights FogFrontL"
  Demux/24 -> BusCreator/24  "VhclCtrl Lights IndR"
  Demux/23 -> BusCreator/23  "VhclCtrl Lights IndL"
  Demux/22 -> BusCreator/22  "VhclCtrl Lights ParkR"
  Demux/21 -> BusCreator/21  "VhclCtrl Lights ParkL"
  Demux/20 -> BusCreator/20  "VhclCtrl Lights Daytime"
  Demux/19 -> BusCreator/19  "VhclCtrl Lights HighBeam"
  Demux/18 -> BusCreator/18  "VhclCtrl Lights LowBeam"
  Demux/17 -> BusCreator/17  "VhclCtrl Steering Trq"
  Demux/16 -> BusCreator/16  "VhclCtrl Steering AngAcc"
  Demux/15 -> BusCreator/15  "VhclCtrl Steering AngVel"
  Demux/14 -> BusCreator/14  "VhclCtrl Steering Ang"
  Demux/13 -> BusCreator/13  "VhclCtrl Gas"
  Demux/12 -> BusCreator/12  "VhclCtrl Clutch"
  Demux/11 -> BusCreator/11  "VhclCtrl BrakePark"
  Demux/10 -> BusCreator/10  "VhclCtrl Brake"
  Demux/9 -> BusCreator/9  "VhclCtrl SelectorCtrl"
  Demux/8 -> BusCreator/8  "VhclCtrl GearNo"
  Demux/7 -> BusCreator/7  "VhclCtrl UserSignal4"
  Demux/6 -> BusCreator/6  "VhclCtrl UserSignal3"
  Demux/5 -> BusCreator/5  "VhclCtrl UserSignal2"
  Demux/4 -> BusCreator/4  "VhclCtrl UserSignal1"
  Demux/3 -> BusCreator/3  "VhclCtrl UserSignal0"
  Demux/2 -> BusCreator/2  "VhclCtrl Key"
  Demux/1 -> BusCreator/1  "VhclCtrl SST"
  BusCreator/1 -> Out/1
  In/1 -> Demux/1

== system generic_truck/TruckMaker/VehicleControl/CreateBus VhclCtrl.PT ==
  In1 : Inport
  BusCreator1 : BusCreator  Inputs=12
  Demux1 : Demux  Outputs=12
      settings: DisplayOption=none
  Out1 : Outport  VectorParamsAs1DForOutWhenUnconnected=off
  wires:
  BusCreator1/1 -> Out1/1
  In1/1 -> Demux1/1
  Demux1/1 -> BusCreator1/1  "VhclCtrl SST"
  Demux1/2 -> BusCreator1/2  "VhclCtrl Key"
  Demux1/3 -> BusCreator1/3  "VhclCtrl UserSignal0"
  Demux1/4 -> BusCreator1/4  "VhclCtrl UserSignal1"
  Demux1/5 -> BusCreator1/5  "VhclCtrl UserSignal2"
  Demux1/6 -> BusCreator1/6  "VhclCtrl UserSignal3"
  Demux1/7 -> BusCreator1/7  "VhclCtrl UserSignal4"
  Demux1/8 -> BusCreator1/8  "VhclCtrl GearNo"
  Demux1/9 -> BusCreator1/9  "VhclCtrl SelectorCtrl"
  Demux1/10 -> BusCreator1/10  "VhclCtrl Clutch"
  Demux1/11 -> BusCreator1/11  "VhclCtrl Gas"
  Demux1/12 -> BusCreator1/12  "VhclCtrl Brake"

== system generic_truck/TruckMaker/VehicleControl/CreateBus VhclCtrl.Steering ==
  In1 : Inport
  Bus Creator : BusCreator  Inputs=5
  Demux : Demux  Outputs=5
      settings: DisplayOption=none
  Out1 : Outport  VectorParamsAs1DForOutWhenUnconnected=off
  wires:
  In1/1 -> Demux/1
  Bus Creator/1 -> Out1/1
  Demux/1 -> Bus Creator/1  "VhclCtrl Steering Ang"
  Demux/5 -> Bus Creator/5  "VhclCtrl Steering ByTrq"
  Demux/3 -> Bus Creator/3  "VhclCtrl Steering AngAcc"
  Demux/2 -> Bus Creator/2  "VhclCtrl Steering AngVel"
  Demux/4 -> Bus Creator/4  "VhclCtrl Steering Trq"

== system generic_truck/TruckMaker/IPG Vehicle/Brake/CreateBus Vhcl.Wheel.PT ==
  In : Inport
  BusCreator : BusCreator  Inputs=60
  Demux : Demux  Outputs=60
      settings: DisplayOption=none
  Out : Outport  VectorParamsAs1DForOutWhenUnconnected=off
  wires:
  Demux/60 -> BusCreator/60  "Vhcl Trq_DriveSrc_trg d11"
  Demux/59 -> BusCreator/59  "Vhcl Trq_DriveSrc_trg d10"
  Demux/58 -> BusCreator/58  "Vhcl Trq_DriveSrc_trg d9"
  Demux/57 -> BusCreator/57  "Vhcl Trq_DriveSrc_trg d8"
  Demux/56 -> BusCreator/56  "Vhcl Trq_DriveSrc_trg d7"
  Demux/55 -> BusCreator/55  "Vhcl Trq_DriveSrc_trg d6"
  Demux/54 -> BusCreator/54  "Vhcl Trq_DriveSrc_trg d5"
  Demux/53 -> BusCreator/53  "Vhcl Trq_DriveSrc_trg d4"
  Demux/52 -> BusCreator/52  "Vhcl Trq_DriveSrc_trg d3"
  Demux/51 -> BusCreator/51  "Vhcl Trq_DriveSrc_trg d2"
  Demux/50 -> BusCreator/50  "Vhcl Trq_DriveSrc_trg d1"
  Demux/49 -> BusCreator/49  "Vhcl Trq_DriveSrc_trg d0"
  Demux/48 -> BusCreator/48  "Vhcl Wheel RR4 WhlBearing"
  Demux/47 -> BusCreator/47  "Vhcl Wheel RR4 Trq_T2W"
  Demux/46 -> BusCreator/46  "Vhcl Wheel RR4 Trq_BrakeReg_trg"
  Demux/45 -> BusCreator/45  "Vhcl Wheel RR4 Trq_Brake"
  Demux/44 -> BusCreator/44  "Vhcl Wheel RL4 WhlBearing"
  Demux/43 -> BusCreator/43  "Vhcl Wheel RL4 Trq_T2W"
  Demux/42 -> BusCreator/42  "Vhcl Wheel RL4 Trq_BrakeReg_trg"
  Demux/41 -> BusCreator/41  "Vhcl Wheel RL4 Trq_Brake"
  Demux/40 -> BusCreator/40  "Vhcl Wheel RR3 WhlBearing"
  Demux/39 -> BusCreator/39  "Vhcl Wheel RR3 Trq_T2W"
  Demux/38 -> BusCreator/38  "Vhcl Wheel RR3 Trq_BrakeReg_trg"
  Demux/37 -> BusCreator/37  "Vhcl Wheel RR3 Trq_Brake"
  Demux/36 -> BusCreator/36  "Vhcl Wheel RL3 WhlBearing"
  Demux/35 -> BusCreator/35  "Vhcl Wheel RL3 Trq_T2W"
  Demux/34 -> BusCreator/34  "Vhcl Wheel RL3 Trq_BrakeReg_trg"
  Demux/33 -> BusCreator/33  "Vhcl Wheel RL3 Trq_Brake"
  Demux/32 -> BusCreator/32  "Vhcl Wheel FR2 WhlBearing"
  Demux/31 -> BusCreator/31  "Vhcl Wheel FR2 Trq_T2W"
  Demux/30 -> BusCreator/30  "Vhcl Wheel FR2 Trq_BrakeReg_trg"
  Demux/29 -> BusCreator/29  "Vhcl Wheel FR2 Trq_Brake"
  Demux/28 -> BusCreator/28  "Vhcl Wheel FL2 WhlBearing"
  Demux/27 -> BusCreator/27  "Vhcl Wheel FL2 Trq_T2W"
  Demux/26 -> BusCreator/26  "Vhcl Wheel FL2 Trq_BrakeReg_trg"
  Demux/25 -> BusCreator/25  "Vhcl Wheel FL2 Trq_Brake"
  Demux/24 -> BusCreator/24  "Vhcl Wheel RR2 WhlBearing"
  Demux/23 -> BusCreator/23  "Vhcl Wheel RR2 Trq_T2W"
  Demux/22 -> BusCreator/22  "Vhcl Wheel RR2 Trq_BrakeReg_trg"
  Demux/21 -> BusCreator/21  "Vhcl Wheel RR2 Trq_Brake"
  Demux/20 -> BusCreator/20  "Vhcl Wheel RL2 WhlBearing"
  Demux/19 -> BusCreator/19  "Vhcl Wheel RL2 Trq_T2W"
  Demux/18 -> BusCreator/18  "Vhcl Wheel RL2 Trq_BrakeReg_trg"
  Demux/17 -> BusCreator/17  "Vhcl Wheel RL2 Trq_Brake"
  Demux/16 -> BusCreator/16  "Vhcl Wheel RR WhlBearing"
  Demux/15 -> BusCreator/15  "Vhcl Wheel RR Trq_T2W"
  Demux/14 -> BusCreator/14  "Vhcl Wheel RR Trq_BrakeReg_trg"
  Demux/13 -> BusCreator/13  "Vhcl Wheel RR Trq_Brake"
  Demux/12 -> BusCreator/12  "Vhcl Wheel RL WhlBearing"
  Demux/11 -> BusCreator/11  "Vhcl Wheel RL Trq_T2W"
  Demux/10 -> BusCreator/10  "Vhcl Wheel RL Trq_BrakeReg_trg"
  Demux/9 -> BusCreator/9  "Vhcl Wheel RL Trq_Brake"
  Demux/8 -> BusCreator/8  "Vhcl Wheel FR WhlBearing"
  Demux/7 -> BusCreator/7  "Vhcl Wheel FR Trq_T2W"
  Demux/6 -> BusCreator/6  "Vhcl Wheel FR Trq_BrakeReg_trg"
  Demux/5 -> BusCreator/5  "Vhcl Wheel FR Trq_Brake"
  Demux/4 -> BusCreator/4  "Vhcl Wheel FL WhlBearing"
  Demux/3 -> BusCreator/3  "Vhcl Wheel FL Trq_T2W"
  Demux/2 -> BusCreator/2  "Vhcl Wheel FL Trq_BrakeReg_trg"
  Demux/1 -> BusCreator/1  "Vhcl Wheel FL Trq_Brake"
  BusCreator/1 -> Out/1
  In/1 -> Demux/1
